simulink model "Ejer9_EstabilidadCI"  (R2023b)
settings: Solver=ode45  StartTime=0  StopTime=10  RelTol=1e-3
undefined symbols (not defined in the file or in its folder): ci
settings Model: Creator=alfre  LastModifiedBy=alfre

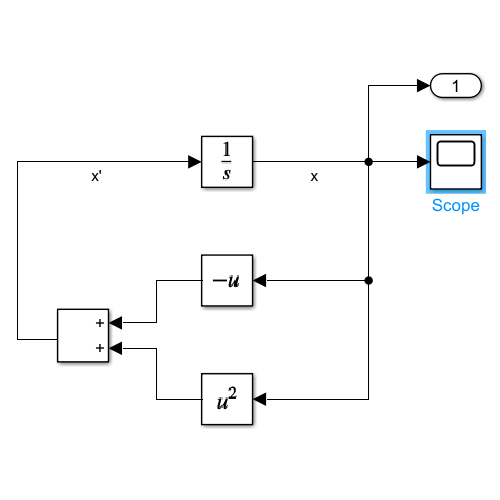
[thumbnail: Simulink's stored preview of the top-level diagram]
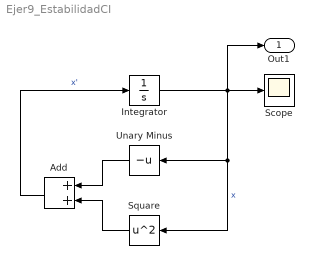
== system Ejer9_EstabilidadCI ==
  Add : Sum
  Integrator : Integrator  InitialCondition=ci
  Scope : Scope
  Square : Math  Operator=square
  Unary Minus : UnaryMinus
  Out1 : Outport
  wires:
  Integrator/1 -> Out1/1, Unary Minus/1, Square/1, Scope/1  "x"
  Unary Minus/1 -> Add/1
  Square/1 -> Add/2
  Add/1 -> Integrator/1  "x'"
